simulink model "PROGRAMMING_EXERCISE_PART11"  (R2017b)
settings: Solver=VariableStepAuto  StartTime=0.0  StopTime=100  RelTol=1e-6
settings Model: Creator=chenjiasheng  LastModifiedBy=chenjiasheng

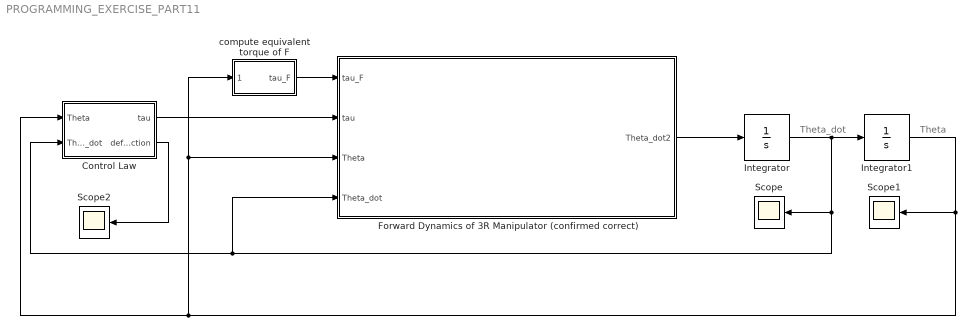
== system PROGRAMMING_EXERCISE_PART11 ==
  note: Theta_dot
  note: Theta
  Control Law : MATLAB Function  TreatAsAtomicUnit=on
  Forward Dynamics of 3R Manipulator (confirmed correct) : MATLAB Function  TreatAsAtomicUnit=on
  Integrator : Integrator  InitialCondition=[0 0 0]'
  Integrator1 : Integrator  InitialCondition=[pi/3 -pi/2 pi/6]'
  Scope : Scope
  Scope1 : Scope
  Scope2 : Scope
  compute equivalent torque of F : MATLAB Function  TreatAsAtomicUnit=on
  wires:
  Forward Dynamics of 3R Manipulator (confirmed correct)/1(Theta_dot2) -> Integrator/1
  Integrator/1 -> Integrator1/1, Scope/1, Control Law/2(Theta_dot), Forward Dynamics of 3R Manipulator (confirmed correct)/4(Theta_dot)
  Integrator1/1 -> Scope1/1, Control Law/1(Theta), compute equivalent torque of F/1(Theta), Forward Dynamics of 3R Manipulator (confirmed correct)/3(Theta)
  compute equivalent torque of F/1(tau_F) -> Forward Dynamics of 3R Manipulator (confirmed correct)/1(tau_F)
  Control Law/1(tau) -> Forward Dynamics of 3R Manipulator (confirmed correct)/2(tau)
  Control Law/2(deflection) -> Scope2/1

== matlab function PROGRAMMING_EXERCISE_PART11/Control Law ==
  data: Theta input; tau output; deflection output; Theta_dot input
function [tau,deflection] = fcn(Theta,Theta_dot)
Theta_d=[pi/3 -pi/2 pi/6]';
Theta_d_dot=[0 0 0]';
Kpx=diag([10 1000 1000]); % 
Kv=diag([100 0 0]);
%%
L1=4;L2=3;L3=2;
theta1=Theta(1);theta2=Theta(2);theta3=Theta(3);
E=Theta_d-Theta;
E_dot=Theta_d_dot-Theta_dot;
J=[L1*sin(theta2+theta3)+L2*sin(theta3)    L2*sin(theta3)    0;
   L1*cos(theta2+theta3)+L2*cos(theta3)+L3 L2*cos(theta3)+L3 L3;
   1                                       1                 1];
tau=J'*Kpx*J*E+Kv*E_dot;
deflection=J*E;
end

== matlab function PROGRAMMING_EXERCISE_PART11/Forward Dynamics of 3R Manipulator (confirmed correct) ==
  data: tau_F input; tau input; Theta_dot2 output; Theta input; Theta_dot input
function Theta_dot2  = fcn(tau_F,tau,Theta,Theta_dot)
L1=4;L2=3;L3=2;
m1=20;m2=15;m3=10;
Izz1=0.5;Izz2=0.2;Izz3=0.1;
theta1=Theta(1);theta2=Theta(2);theta3=Theta(3);
theta1_dot=Theta_dot(1);theta2_dot=Theta_dot(2);theta3_dot=Theta_dot(3);
g=9.81;
M=zeros(3);
M(1,1)=(1/4*m1+m2+m3)*L1^2+(1/4*m2+m3)*L2^2+(m2+2*m3)*L1*L2*cos(theta2)+1/4*m3*L3^2+m3*L1*L3*cos(theta2+theta3)+m3*L2*L3*cos(theta3)+Izz1+Izz2+Izz3;
M(1,2)=(1/4*m2+m3)*L2^2+(1/2*m2+m3)*L1*L2*cos(theta2)+1/4*m3*L3^2+1/2*m3*L1*L3*cos(theta2+theta3)+m3*L2*L3*cos(theta3)+Izz2+Izz3;
M(1,3)=1/4*m3*L3^2+1/2*m3*L1*L3*cos(theta2+theta3)+1/2*m3*L2*L3*cos(theta3)+Izz3;
M(2,1)=m3*L2*L3*cos(theta3)+(1/4*m2+m3)*L2^2+(1/2*m2+m3)*L1*L2*cos(theta2)+1/4*m3*L3^2+1/2*m3*L1*L3*cos(theta2+theta3)+Izz2+Izz3;
M(2,2)=m3*L2*L3*cos(theta3)+(1/4*m2+m3)*L2^2+1/4*m3*L3^2+Izz2+Izz3;
M(2,3)=m3/2*L2*L3*cos(theta3)+1/4*m3*L3^2+Izz3;
M(3,1)=1/4*m3*L3^2+m3/2*L1*L3*cos(theta2+theta3)+m3/2*L2*L3*cos(theta3)+Izz3;
M(3,2)=1/4*m3*L3^2+m3/2*L2*L3*cos(theta3)+Izz3;
M(3,3)=1/4*m3*L3^2+Izz3;
V=zeros(3,1);
V(1)=-(1/2*m2+m3)*L1*L2*sin(theta2)*theta2_dot*(2*theta1_dot+theta2_dot)-1/2*m3*L1*L3*sin(theta2+theta3)*(theta2_dot+theta3_dot)*(2*theta1_dot+theta2_dot+theta3_dot)-1/2*m3*L2*L3*sin(theta3)*theta3_dot*(2*theta1_dot+2*theta2_dot+theta3_dot)
V(2)=(1/2*m2+m3)*L1*L2*sin(theta2)*theta1_dot^2+1/2*m3*L1*L3*sin(theta2+theta3)*theta1_dot^2+1/2*m3*L2*L3*(-sin(theta3)*theta3_dot*(2*theta1_dot+2*theta2_dot+theta3_dot))
V(3)=1/2*m3*(L1*L3*sin(theta2+theta3)*theta1_dot^2+L2*L3*sin(theta3)*(theta1_dot+theta2_dot)^2)

%% gravitational term
G=zeros(3,1);
% G(1)=m1*g*L1/2*cos(theta1)+m2*g*(L1*cos(theta1)+L2/2*cos(theta1+theta2))+m3*g*(L1*cos(theta1)+L2*cos(theta1+theta2)+L3/2*cos(theta1+theta2+theta3))
% G(2)=m2*g*L2/2*cos(theta1+theta2)+m3*g*(L2*cos(theta1+theta2)+L3/2*cos(theta1+theta2+theta3))
% G(3)=m3*g*L3/2*cos(theta1+theta2+theta3)
%% output
tau=tau+tau_F;
Theta_dot2=inv(M)*(tau-V-G);
end

== matlab function PROGRAMMING_EXERCISE_PART11/compute equivalent torque of F ==
  data: Theta input; tau_F output
function tau_F = fcn(Theta)
%%
F=[1 0 0]';
% F=[0 1 0]';
%%
L1=4;L2=3;L3=2;
theta1=Theta(1);theta2=Theta(2);theta3=Theta(3);
J=[L1*sin(theta2+theta3)+L2*sin(theta3)    L2*sin(theta3)    0;
   L1*cos(theta2+theta3)+L2*cos(theta3)+L3 L2*cos(theta3)+L3 L3;
   1                                       1                 1];
%%
tau_F=J'*F
end
